simulink model "IDFT_Ex2"  (R2023a)
settings: Solver=VariableStepAuto  StartTime=0.0  StopTime=0.1  RelTol=1e-3
undefined symbols (not defined in the file): None, S, vsva2197, xcvc1902
libraries: dspsrcs4 x1, aieDSP x1, vmcUtilities x1
settings Model: Creator=sdegala  LastModifiedBy=robg
settings ModelReferenceCC: EnableRefExpFcnMdlSchedulingChecks=on

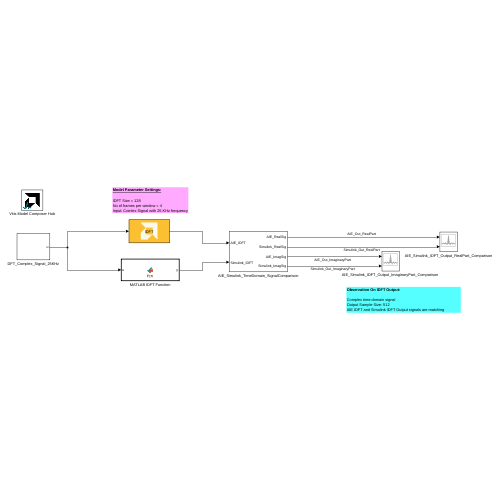
[thumbnail: Simulink's stored preview of the top-level diagram]
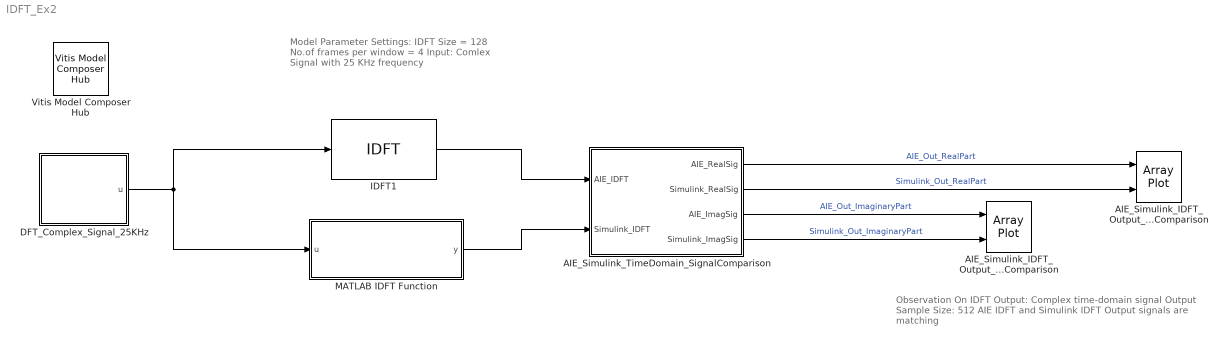
== system IDFT_Ex2 ==
  note: Model Parameter Settings:
      |
      | IDFT Size = 128
      | No.of frames per window = 4
      | Input: Comlex Signal with 25 KHz frequency
  note: Observation On IDFT Output:
      |
      | Complex time-domain signal
      | Output Sample Size: 512
      | AIE IDFT and Simulink IDFT Output signals are matching
  "AIE_Simulink_IDFT_Output_ImaginaryPart_Comparison " : ArrayPlot  NumInputPorts=2  WindowPosition=[2.000000,37.000000,1280.000000,655.000000,]  PlotType=Line  AxesScaling=Manual  YLimits=[-180,180]  ShowLegend=on
  AIE_Simulink_IDFT_Output_RealPart_Comparison : ArrayPlot  NumInputPorts=2  WindowPosition=[2.000000,37.000000,1280.000000,655.000000,]  PlotType=Line  YLimits=[-159.9998,159.9998]  ShowLegend=on
  AIE_Simulink_TimeDomain_SignalComparison : Subsystem
  DFT_Complex_Signal_25KHz : Subsystem
  IDFT1 : aieDSP/IDFT  data_type=cfloat  twiddle_type=cfloat  point_size=128  num_frames=4  shift_val=0  rnd_mode=Round symmetrical to infinity  ssr=1  sat_mode=0-None  casc_length=1  AIE_VARIANT=1  blockJsonConstraints=[]  blockJsonConstraintsInternal=[]  spec=vmc_idft.json  SerializedMaskParamNames=[]  SerializedMaskParamValues=[]  SerializedMaskParamVisibilities=[]  block_type=IDFT  SerializedMaskParamDataypes=typename|typename|uint|uint|uint|uint|uint|uint|uint|uint  SerializedMaskParamEnumStrArr=0|0|0|0|0|Floor,Ceiling,Round to positive infinity,Round to negative infinity,Round symmetrical to infinity,Round symmetrical to zero,Round convergent to even,Round convergent to odd|0|0-None,1-Asymmetric,3-Symmetric|0|0  SerializedMaskParamEnumValArr=0|0|0|0|0|0,1,2,3,4,5,6,7|0|0,1,3|0|0  SerializedMaskParamVectorArr=0|0|0|0|0|0|0|0|0|0
  MATLAB IDFT Function : MATLAB Function  TreatAsAtomicUnit=on
  Vitis Model Composer Hub : vmcUtilities/Vitis Model Composer Hub  Tag=genX  CodeGeneration=off  SubsystemName=AIE_Subsystem  StartColumn=1  NumberOfColumns=1  TargetDirectory=./code  exportDesign=off  analyzeDesign=off  validateDesignOnHw=off  ExportType=AI Engines  IpVendor=xilinx.com  IpLibrary=hls  IpVersion=1.0  IpHWLanguage=Verilog  AieCompilerOptions={}  AieSimulatorOptions={}  CreateTestbench=off  TestbenchStackSize=10  RunRtlSim=off  RunCSim=off  RunAieSim=off  AieSimTimeout=50000  RunAieSimProfiling=off  LaunchVitisAnalyzer=off  PlotOutput=off  RunX86Sim=off  X86SimTimeout=10  GenHwImage=off  GenLibadfXo=off  GenHwValidationCode=off  PlatformType=Not Specified  HwSystemType=Baremetal  HwValidationTarget=hw  ProjDevice=xcvc1902-vsva2197-1LP-e-S  ProjDevicePart=xcvc1902-vsva2197-1LP-e-S  AIEType=AIE  SamplePeriod=-1  ClockFrequency=200  DataPathParallelism=1  xilinxfamily=versalaicore  part=xcvc1902  speed=-1LP-e-S  package=vsva2197  directory=./netlist  testbench=off  incr_netlist=off  synthesis_tool=Vivado  clock_wrapper=Clock Enables  dbl_ovrd=According to Block Masks  dcm_input_clock_period=10  sysclk_period=10  simulink_period=1  eval_field=0  IPInfoJsonString="{\"AIESubsystem\":{\"SubsystemName\":\"AIE_Subsystem\",\"TargetDirectory\":\"./code\",\"SubsystemDir\":\"./code/ip/AIE_Subsystem\"}}"  LogFileName=/proj/xhdhdstaff5/sdegala/Head1/HEAD/AIE_Block_Examples/AIE/code/model_composer.log  NThreads=4
  wires:
  AIE_Simulink_TimeDomain_SignalComparison/4(Simulink_ImagSig) -> "AIE_Simulink_IDFT_Output_ImaginaryPart_Comparison "/2  "Simulink_Out_ImaginaryPart"
  AIE_Simulink_TimeDomain_SignalComparison/1(AIE_RealSig) -> AIE_Simulink_IDFT_Output_RealPart_Comparison/1  "AIE_Out_RealPart"
  MATLAB IDFT Function/1(y) -> AIE_Simulink_TimeDomain_SignalComparison/2(Simulink_IDFT)
  IDFT1/1 -> AIE_Simulink_TimeDomain_SignalComparison/1(AIE_IDFT)
  DFT_Complex_Signal_25KHz/1(u) -> MATLAB IDFT Function/1(u), IDFT1/1
  AIE_Simulink_TimeDomain_SignalComparison/2(Simulink_RealSig) -> AIE_Simulink_IDFT_Output_RealPart_Comparison/2  "Simulink_Out_RealPart"
  AIE_Simulink_TimeDomain_SignalComparison/3(AIE_ImagSig) -> "AIE_Simulink_IDFT_Output_ImaginaryPart_Comparison "/1  "AIE_Out_ImaginaryPart"

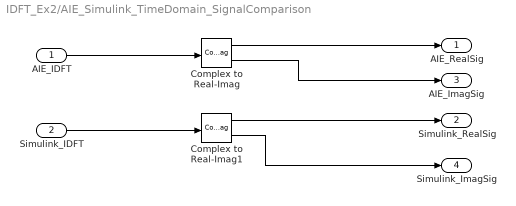
== system IDFT_Ex2/AIE_Simulink_TimeDomain_SignalComparison ==
  AIE_IDFT : Inport
  Simulink_IDFT : Inport  Port=2
  Complex to Real-Imag : ComplexToRealImag
  Complex to Real-Imag1 : ComplexToRealImag
  AIE_RealSig : Outport
  Simulink_RealSig : Outport  Port=2
  AIE_ImagSig : Outport  Port=3
  Simulink_ImagSig : Outport  Port=4
  wires:
  AIE_IDFT/1 -> Complex to Real-Imag/1
  Complex to Real-Imag/1 -> AIE_RealSig/1
  Complex to Real-Imag1/1 -> Simulink_RealSig/1
  Complex to Real-Imag1/2 -> Simulink_ImagSig/1
  Complex to Real-Imag/2 -> AIE_ImagSig/1
  Simulink_IDFT/1 -> Complex to Real-Imag1/1

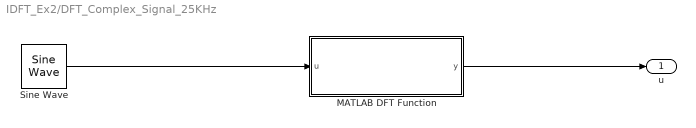
== system IDFT_Ex2/DFT_Complex_Signal_25KHz ==
  MATLAB DFT Function : MATLAB Function  TreatAsAtomicUnit=on
  Sine Wave : dspsrcs4/Sine Wave  Amplitude=1  Frequency=25e3  Phase=0  SampleMode=Discrete  OutComplex=Complex  CompMethod=Trigonometric fcn  TableSize=Speed  SampleTime=1/100e3  SamplesPerFrame=128  ResetState=Restart at time zero  OutputFrames=off  dataType=single  wordLen=16  udDataType=sfix(16)  fracBitsMode=Best precision  numFracBits=15  OutDataTypeStr=single  LastOutDataTypeStr=single
  u : Outport
  wires:
  Sine Wave/1 -> MATLAB DFT Function/1(u)
  MATLAB DFT Function/1(y) -> u/1

== matlab function IDFT_Ex2/MATLAB IDFT Function ==
  data: u input; y output

function y = fcn(u)

IDFT_Size = 128; % IDFT Size
FramesPerWindow = 4; %No.of Frames Per Window

X = single(complex(zeros(IDFT_Size,FramesPerWindow)));

for m = 1:1:FramesPerWindow

     for n = 0:IDFT_Size-1
        for k = 0:IDFT_Size-1
        X(n+1,m) = X(n+1,m) + (u(k+1)*exp(1i*2*pi*n*k/IDFT_Size));
        end
        
     end
        
end

y = (reshape(X,IDFT_Size*FramesPerWindow,1));

== matlab function IDFT_Ex2/DFT_Complex_Signal_25KHz/MATLAB DFT Function ==
  data: u input; y output

function y = fcn(u)

DFT_Size = 128; % DFT Size
FramesPerWindow = 1; %No.of Frames Per Window
u = single(u);

X = single(complex(zeros(DFT_Size,FramesPerWindow)));

for m = 1:1:FramesPerWindow
for k = 0:DFT_Size-1
    for n = 0:DFT_Size-1
        X(k+1,m) = X(k+1,m) + u(n+1)*exp(-1i*2*pi*n*k/DFT_Size);
    end
end
end

y = reshape(X,DFT_Size*FramesPerWindow,1);
